simulink model "ArduCopter_PIDcontrol"  (R2014a)
settings: Solver=FixedStepDiscrete  SolverMode=SingleTasking  StartTime=0.0  StopTime=inf  FixedStep=0.02  RelTol=1e-3
values from neighbouring files (symbols this model uses):
  a = 0.92    [SystemModelParameters.m]
  b = 0.5    [SystemModelParameters.m]
  kd = 50    [SystemModelParameters.m]
  kp = 50    [SystemModelParameters.m]
  L = 284.84*10^-3    (= 0.28484)    [SystemModelParameters.m]
libraries: RC_Library x2, Discrete_IO_Library x2, Timing_Library x2, IMU_Library x1, Serial_Library x1
settings Model: ExtModeTrigDuration=2  Creator=dami  LastModifiedBy=lorem
settings OptimizationCC: OptimizeModelRefInitCode=on  LifeSpan=1  SimCompilerOptimization=On
settings DebuggingCC: UnderspecifiedInitializationDetection=Classic  SolverPrmCheckMsg=none  StateNameClashWarn=warning
settings HardwareCC: ProdBitPerInt=16  ProdBitPerPointer=8  ProdIntDivRoundTo=Zero  ProdEndianess=LittleEndian  ProdWordSize=8  ProdHWDeviceType=Atmel->AVR
settings RTWCC: SystemTargetFile=realtime.tlc  GenerateMakefile=off  TemplateMakefile=realtime.tmf  Description=Run on Target Hardware  RTWVerbose=off  ProcessScript=realtime_make_rtw_hook
settings STFCustomTargetCC: TargetLibSuffix=.a  GenerateSampleERTMain=on  ConcurrentExecutionCompliant=off  GeneratePreprocessorConditionals=Use local settings  ERTCustomFileBanners=on  SupportNonInlinedSFcns=off  SupportVariableSizeSignals=on  MATLABClassNameForMDSCustomization=Simulink.SoftwareTarget.ERTCustomization  GRTInterface=off  SystemTargetFile=realtime.tlc
settings ERTTargetCC: CombineOutputUpdateFcns=off  SupportContinuousTime=on  SupportVariableSizeSignals=on  ExtModeTransport=3  ExtModeMexFile=ext_serial_win32_comm  ExtModeMexArgs=0 1 9600  ERTSrcFileBannerTemplate=realtime_code_template.cgt  ERTHdrFileBannerTemplate=realtime_code_template.cgt  ERTDataSrcFileTemplate=realtime_code_template.cgt  ERTDataHdrFileTemplate=realtime_code_template.cgt  ERTCustomFileTemplate=realtime_file_process.tlc

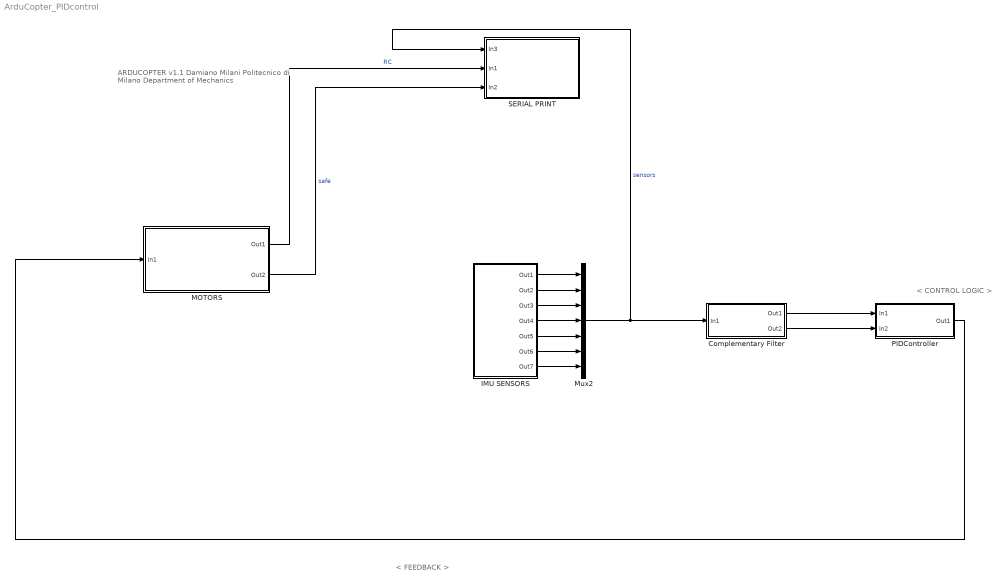
== system ArduCopter_PIDcontrol ==
  note: < CONTROL LOGIC >
  note: ARDUCOPTER v1.1
      |
      | Damiano Milani
      | Politecnico di Milano
      | Department of Mechanics
  note: < FEEDBACK >
  Complementary Filter : Subsystem  ClipboardFcn=""
  "IMU SENSORS " : Subsystem
      settings: AttributesFormatString=6 DOF IMU\nSensors measurements from ArduCopter IMU:\n- 3-axial gyro\n- 3-axial accelerometer\n- temp sensor
  "MOTORS " : Subsystem
      settings: AttributesFormatString=MOTORS ACTUATION WITH SAFE MODE\nIf the safe switch on the RC is armed, it passes the input signal to the 4 motors (red LED).\nIf the safety mode is enabled, the motors are controlled by the RC (blue LED).\nIf an overrun occurs yellow LED is on.\nINPUT: actuation signals [4] from control logic\nOUTPUT: command signals [4] from RC and safe flag [1]
  Mux2 : Mux  Inputs=7
  PIDController : Subsystem
  "SERIAL PRINT " : Subsystem
      settings: AttributesFormatString=DATA TRANSMISSION\nData transmission to serial port:\n(deactivate if overrun occurs)\n- elapsed time [1]\n- real time [1]\n- IMU sensors [7]\n- RC signals [4]\n- safe mode [1]
  wires:
  "MOTORS "/1(Out1) -> "SERIAL PRINT "/2(In1)  "RC"
  "MOTORS "/2(Out2) -> "SERIAL PRINT "/3(In2)  "safe"
  Mux2/1 -> "SERIAL PRINT "/1(In3), Complementary Filter/1(In1)  "sensors"
  "IMU SENSORS "/1(Out1) -> Mux2/1
  "IMU SENSORS "/2(Out2) -> Mux2/2
  "IMU SENSORS "/3(Out3) -> Mux2/3
  "IMU SENSORS "/4(Out4) -> Mux2/4
  "IMU SENSORS "/5(Out5) -> Mux2/5
  "IMU SENSORS "/6(Out6) -> Mux2/6
  "IMU SENSORS "/7(Out7) -> Mux2/7
  Complementary Filter/1(Out1) -> PIDController/1(In1)
  Complementary Filter/2(Out2) -> PIDController/2(In2)
  PIDController/1(Out1) -> "MOTORS "/1(In1)

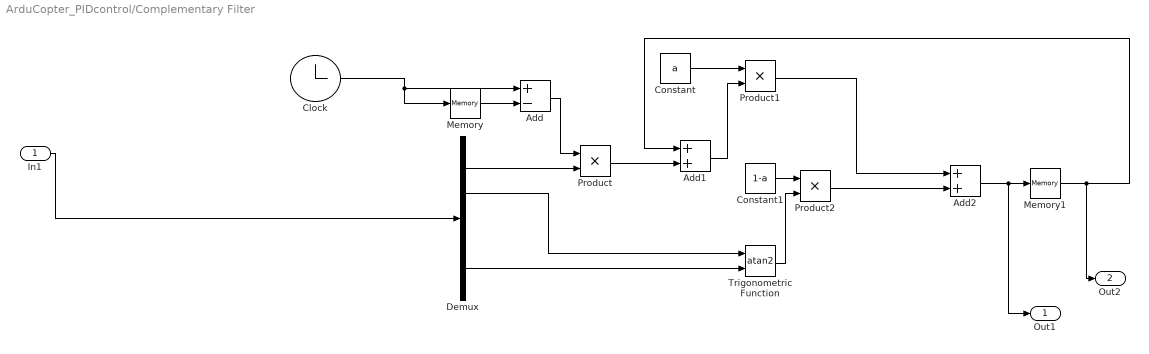
== system ArduCopter_PIDcontrol/Complementary Filter ==
  In1 : Inport
  Add : Sum  Inputs=+-
  Add1 : Sum
  Add2 : Sum
  Clock : Clock
  Constant : Constant  Value=a
  Constant1 : Constant  Value=1-a
  Demux : Demux  Outputs=7
  Memory : Memory  InheritSampleTime=on
  Memory1 : Memory  InheritSampleTime=on
  Product : Product
  Product1 : Product
  Product2 : Product
  Trigonometric Function : Trigonometry  Operator=atan2
  Out1 : Outport
  Out2 : Outport  Port=2
  wires:
  In1/1 -> Demux/1
  Demux/3 -> Trigonometric Function/1
  Demux/6 -> Trigonometric Function/2
  Clock/1 -> Memory/1, Add/1
  Memory/1 -> Add/2
  Demux/2 -> Product/2
  Add/1 -> Product/1
  Product/1 -> Add1/2
  Add1/1 -> Product1/2
  Constant/1 -> Product1/1
  Trigonometric Function/1 -> Product2/2
  Constant1/1 -> Product2/1
  Product2/1 -> Add2/2
  Product1/1 -> Add2/1
  Add2/1 -> Out1/1, Memory1/1
  Memory1/1 -> Out2/1, Add1/1

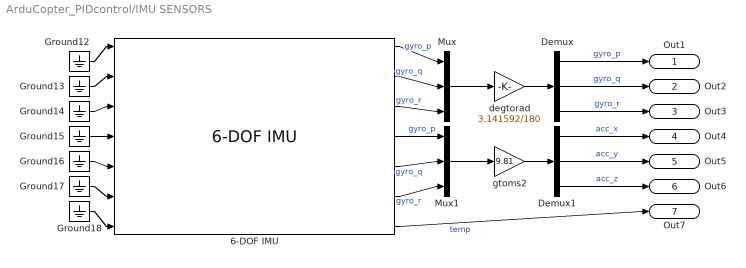
== system ArduCopter_PIDcontrol/IMU SENSORS  ==
  " 6-DOF IMU " : IMU_Library/6-DOF IMU  lpf_filt_freq_hz_ix=20 Hz  gyro_scale_ix=+/- 500 deg/sec  accel_scale_ix=+/- 8g  SampleTime=0.02  lpf_filt_freq_hz=5 Hz  gyro_scale=+/- 250 deg/sec  accel_scale=+/- 2g
  Demux : Demux  Outputs=3
  Demux1 : Demux  Outputs=3
  Ground{12..18} (7 alike) : Ground
  Mux : Mux  Inputs=3
  Mux1 : Mux  Inputs=3
  degtorad : Gain  Gain=3.141592/180
  gtoms2 : Gain  Gain=9.81
  Out1 : Outport
  Out2 : Outport  Port=2
  Out3 : Outport  Port=3
  Out4 : Outport  Port=4
  Out5 : Outport  Port=5
  Out6 : Outport  Port=6
  Out7 : Outport  Port=7
  wires:
  Ground13/1 -> " 6-DOF IMU "/2
  Ground12/1 -> " 6-DOF IMU "/1
  Ground15/1 -> " 6-DOF IMU "/4
  Ground14/1 -> " 6-DOF IMU "/3
  Demux/1 -> Out1/1  "gyro_p"
  Ground17/1 -> " 6-DOF IMU "/6
  Demux/3 -> Out3/1  "gyro_r"
  Demux1/2 -> Out5/1  "acc_y"
  Ground16/1 -> " 6-DOF IMU "/5
  Demux1/3 -> Out6/1  "acc_z"
  Demux1/1 -> Out4/1  "acc_x"
  " 6-DOF IMU "/7 -> Out7/1  "temp"
  Ground18/1 -> " 6-DOF IMU "/7
  Demux/2 -> Out2/1  "gyro_q"
  degtorad/1 -> Demux/1
  gtoms2/1 -> Demux1/1
  Mux/1 -> degtorad/1
  " 6-DOF IMU "/1 -> Mux/1  "gyro_p"
  " 6-DOF IMU "/2 -> Mux/2  "gyro_q"
  " 6-DOF IMU "/3 -> Mux/3  "gyro_r"
  Mux1/1 -> gtoms2/1
  " 6-DOF IMU "/4 -> Mux1/1  "gyro_p"
  " 6-DOF IMU "/5 -> Mux1/2  "gyro_q"
  " 6-DOF IMU "/6 -> Mux1/3  "gyro_r"

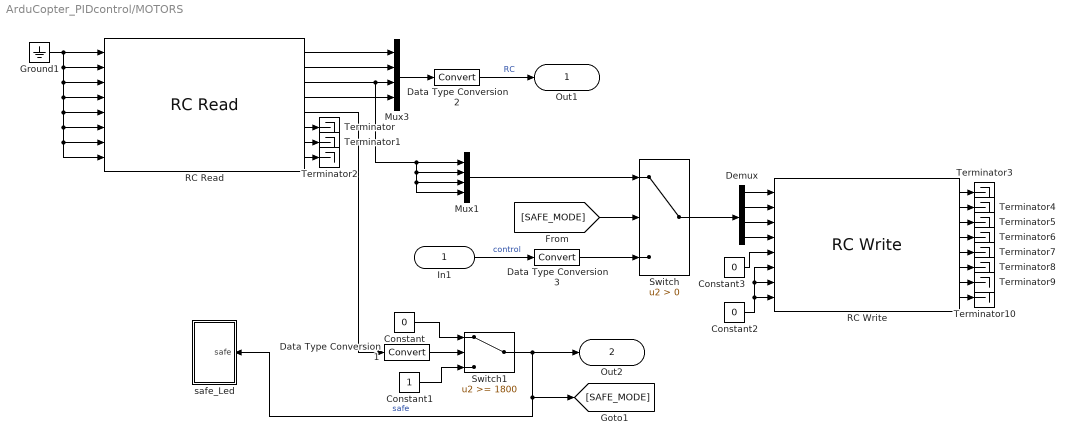
== system ArduCopter_PIDcontrol/MOTORS  ==
  In1 : Inport  Description=4 signals for the motors FROM CONTROL
  Constant : Constant  Value=0  OutDataTypeStr=int8
  Constant1 : Constant  OutDataTypeStr=int8
  Constant2 : Constant  Value=0  OutDataTypeStr=uint16
  Constant3 : Constant  Value=0  OutDataTypeStr=int16
  Data Type Conversion1 : DataTypeConversion
  Data Type Conversion2 : DataTypeConversion
  Data Type Conversion3 : DataTypeConversion
  Demux : Demux
  Ground1 : Ground
  Mux1 : Mux
  Mux3 : Mux
  RC Read : RC_Library/RC Read
  RC Write : RC_Library/RC Write
  Switch : Switch  Criteria=u2 > Threshold
  Switch1 : Switch  Threshold=1800
  Terminator{,1..10} (11 alike) : Terminator
  safe_Led : Subsystem
  Out1 : Outport
  Out2 : Outport  Port=2
  wires:
  Demux/1 -> RC Write/1
  Demux/4 -> RC Write/4
  Demux/2 -> RC Write/2
  Demux/3 -> RC Write/3
  Switch/1 -> Demux/1
  [SAFE_MODE] -> Switch/2
  RC Write/4 -> Terminator6/1
  RC Write/5 -> Terminator7/1
  RC Write/6 -> Terminator8/1
  Data Type Conversion2/1 -> Out1/1  "RC"
  Mux3/1 -> Data Type Conversion2/1
  Ground1/1 -> RC Read/5, RC Read/6, RC Read/7, RC Read/8, RC Read/4, RC Read/3, RC Read/2, RC Read/1
  RC Read/2 -> Mux3/2
  RC Read/4 -> Mux3/4
  RC Read/1 -> Mux3/1
  RC Write/3 -> Terminator5/1
  RC Write/1 -> Terminator3/1
  RC Read/3 -> Mux1/4, Mux1/3, Mux1/2, Mux1/1, Mux3/3
  RC Write/2 -> Terminator4/1
  RC Read/8 -> Terminator2/1
  RC Write/8 -> Terminator10/1
  RC Write/7 -> Terminator9/1
  RC Read/7 -> Terminator1/1
  RC Read/6 -> Terminator/1
  In1/1 -> Data Type Conversion3/1  "control"
  Data Type Conversion3/1 -> Switch/3
  Mux1/1 -> Switch/1
  Data Type Conversion1/1 -> Switch1/2
  Constant1/1 -> Switch1/3
  Constant/1 -> Switch1/1
  RC Read/5 -> Data Type Conversion1/1
  Switch1/1 -> safe_Led/1(safe), [SAFE_MODE], Out2/1  "safe"
  Constant2/1 -> RC Write/6, RC Write/7, RC Write/8
  Constant3/1 -> RC Write/5

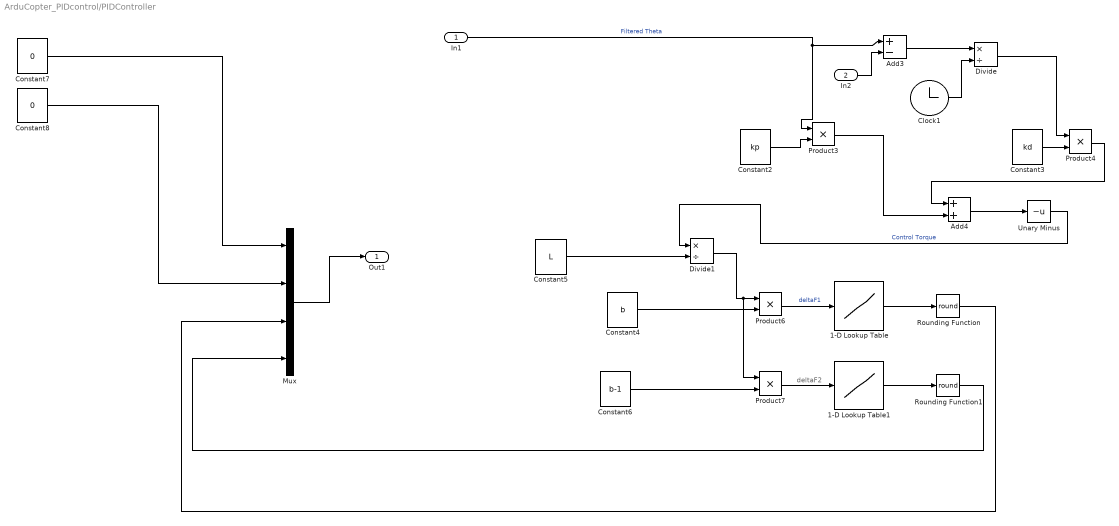
== system ArduCopter_PIDcontrol/PIDController ==
  note: deltaF2
  In1 : Inport
  In2 : Inport  Port=2
  1-D Lookup Table : Lookup_n-D  NumberOfTableDimensions=1  BreakpointsForDimension1=[-2,2]  Table=[1447,1792]  InternalRulePriority=Speed  RndMeth=Simplest  InputSameDT=on
  1-D Lookup Table1 : Lookup_n-D  NumberOfTableDimensions=1  BreakpointsForDimension1=[-2,2]  Table=[1455,1832]  InternalRulePriority=Speed  RndMeth=Simplest  InputSameDT=on
  Add3 : Sum  Inputs=+-
  Add4 : Sum
  Clock1 : Clock
  Constant2 : Constant  Value=kp
  Constant3 : Constant  Value=kd
  Constant4 : Constant  Value=b
  Constant5 : Constant  Value=L
  Constant6 : Constant  Value=b-1
  Constant7 : Constant  Value=0
  Constant8 : Constant  Value=0
  Divide : Product  Inputs=*/
  Divide1 : Product  Inputs=*/
  Mux : Mux
  Product{3..4,6..7} (4 alike) : Product
  Rounding Function : Rounding  Operator=round
  Rounding Function1 : Rounding  Operator=round
  Unary Minus : UnaryMinus
  Out1 : Outport
  wires:
  In1/1 -> Product3/1, Add3/1  "Filtered Theta"
  Add3/1 -> Divide/1
  Clock1/1 -> Divide/2
  Constant2/1 -> Product3/2
  Divide/1 -> Product4/1
  Constant3/1 -> Product4/2
  Product4/1 -> Add4/1
  Product3/1 -> Add4/2
  Add4/1 -> Unary Minus/1
  Unary Minus/1 -> Divide1/1  "Control Torque"
  Constant5/1 -> Divide1/2
  Divide1/1 -> Product7/1, Product6/1
  Constant4/1 -> Product6/2
  Constant6/1 -> Product7/2
  Product6/1 -> 1-D Lookup Table/1  "deltaF1"
  Product7/1 -> 1-D Lookup Table1/1
  1-D Lookup Table/1 -> Rounding Function/1
  1-D Lookup Table1/1 -> Rounding Function1/1
  Rounding Function/1 -> Mux/3
  Rounding Function1/1 -> Mux/4
  In2/1 -> Add3/2
  Constant8/1 -> Mux/2
  Constant7/1 -> Mux/1
  Mux/1 -> Out1/1

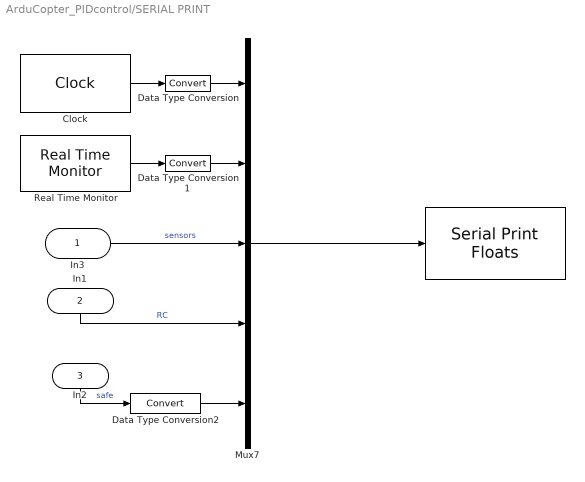
== system ArduCopter_PIDcontrol/SERIAL PRINT  ==
  In3 : Inport
  In1 : Inport  Port=2
  In2 : Inport  Port=3
  " " : Serial_Library/Serial Print Floats  baud=57600  uart=UART0  SampleTime=-1
  Clock : Timing_Library/Clock  SampleTime=.02
  Data Type Conversion : DataTypeConversion
  Data Type Conversion1 : DataTypeConversion
  Data Type Conversion2 : DataTypeConversion
  Mux7 : Mux  Inputs=5
  Real Time Monitor : Timing_Library/Real Time Monitor  SampleTime=0.02
  wires:
  In3/1 -> Mux7/3  "sensors"
  Data Type Conversion/1 -> Mux7/1
  Real Time Monitor/1 -> Data Type Conversion1/1
  Clock/1 -> Data Type Conversion/1
  Mux7/1 -> " "/1
  Data Type Conversion1/1 -> Mux7/2
  In2/1 -> Data Type Conversion2/1  "safe"
  In1/1 -> Mux7/4  "RC"
  Data Type Conversion2/1 -> Mux7/5

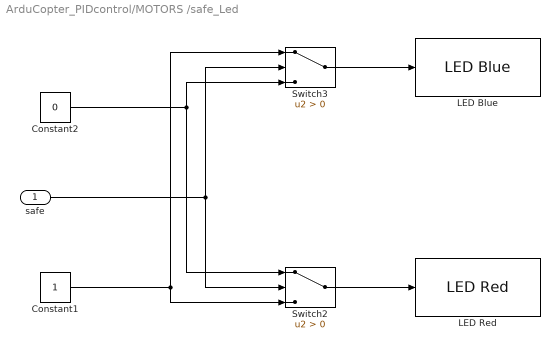
== system ArduCopter_PIDcontrol/MOTORS /safe_Led ==
  safe : Inport
  Constant1 : Constant
  Constant2 : Constant  Value=0
  LED Blue : Discrete_IO_Library/LED Blue
  LED Red : Discrete_IO_Library/LED Red
  Switch2 : Switch  Criteria=u2 > Threshold
  Switch3 : Switch  Criteria=u2 > Threshold
  wires:
  Constant1/1 -> Switch3/1, Switch2/3
  Constant2/1 -> Switch3/3, Switch2/1
  Switch3/1 -> LED Blue/1
  Switch2/1 -> LED Red/1
  safe/1 -> Switch2/2, Switch3/2
